simulink model "CC_dynamic_case"  (R2020b)
settings: Solver=VariableStepAuto  StartTime=0.0  StopTime=3600*2000  RelTol=1e-3
undefined symbols (not defined in the file or in its folder): Batt, BatteryCback, BatteryLoadFcn, gcbh, I_charge, I_discharge, Q, sps_rtmsupport
libraries: simulink x6, powerlib x5
settings Model: SimulationMode=rapid-accelerator  Creator=JIAHANG001  LastModifiedBy=jiahang001
settings SFSimCC: CustomCodeUndefinedFunction=UseInterfaceOnly

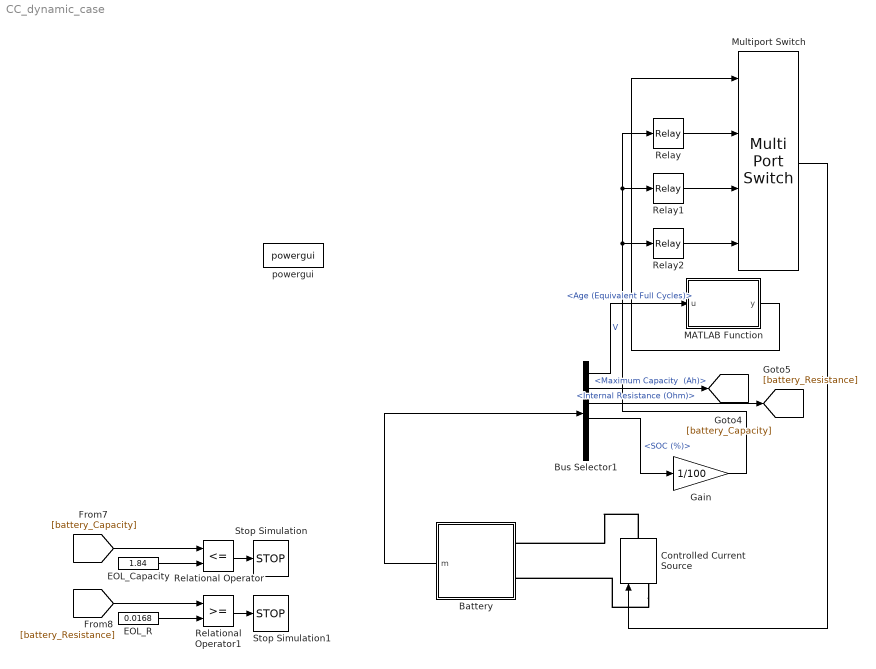
== system CC_dynamic_case ==
  Battery : Subsystem  AncestorBlock=electricdrivelib/Extra Sources/Battery  DialogController=POWERSYS.PowerSysDialog  LoadFcn=sps_rtmsupport('LoadFcn',gcbh); BatteryLoadFcn(gcb)  InitFcn=BatteryCback(gcb,1)  StartFcn=sps_rtmsupport('StartFcn',gcbh);  StopFcn=sps_rtmsupport('StopFcn',gcbh);  mask(Battery){BatType=Lithium-Ion, ShowTempParam=off, ThermalPreset=3.3V  2.3Ah  (LiFePO4), ShowAgeParam=on, NomV=3.3, NomQ=2.3, SOC=100, Batt_Tr=30, PresetModel=off, MaxQ=2.3, MinV=2.475, FullV=3.748, Dis_rate=2.3, R=0.014, Normal_OP=2.25, expZone=[3.4788       0.113], current=[0.15 1.3 3.25], Units=Ampere-hour, Tci=25, NomT=25, T2=0, MaxQ2=2.208, FullV2=3.45, Normal_OP2=2.85, expZone2=[3.22       0.015], Rca=0.6, ti=1000, Dp=0, Neq0=0, Tsim=60, Ta1=25, Qeol=2.3*0.8, Reol=0.014*1.2, Char_age=[2.3, 4.3], Dis_age=[2.3, 11.7], N1=1000, N2=1200, N3=400, N4=500, Ta2=45, N5=950}
      mask prompts: BatType "Type:"; ShowTempParam "Simulate temperature effects"; ThermalPreset "Use a preset battery:"; ShowAgeParam "Simulate aging effects"; NomV "Nominal voltage (V)"; NomQ "Rated capacity (Ah)"; SOC "Initial state-of-charge (%)"; Batt_Tr "Battery response time (s)"; PresetModel "Determined from the nominal parameters of the battery"; MaxQ "Maximum capacity (Ah)"; MinV "Cut-off Voltage (V)"; FullV "Fully charged voltage (V)"; Dis_rate "Nominal discharge current (A)"; R "Internal resistance (Ohms)"; Normal_OP "Capacity (Ah) at nominal voltage"; expZone "Exponential zone [Voltage (V), Capacity (Ah)]"; current "Discharge current [i1, i2, i3,...] (A)"; Tci "Initial cell temperature (deg. C)"; NomT "Nominal ambient temperature T1 (deg. C)"; T2 "Second ambient temperature T2 (deg. C)"; MaxQ2 "Maximum capacity (Ah)"; FullV2 "Initial discharge voltage (V)"; Normal_OP2 "Voltage at 90% maximum capacity (V)"; expZone2 "Exponential zone [Voltage (V), Capacity (Ah)]"; Rca "Thermal resistance, cell-to-ambient (deg. C/W)"; ti "Thermal time constant, cell-to-ambient (s)"; Dp "Heat loss difference [charge vs. discharge] (W)"; Neq0 "Initial battery age (Equivalent full cycles)"; Tsim "Aging model sampling time (s)"; Ta1 "Ambient temperature Ta1 (deg. C)"; Qeol "Capacity at EOL (End Of Life) (Ah)"; Reol "Internal resistance at EOL (Ohms)"; Char_age "Charge current (nominal, maximum) [Ic (A), Icmax (A)]"; Dis_age "Discharge current (nominal, maximum) [Id (A), Idmax (A)]"; N1 "Cycle life at 100 % DOD, Ic and Id (Cycles)"; N2 "Cycle life at 25 % DOD, Ic and Id (Cycles)"; N3 "Cycle life at 100 % DOD, Ic and Idmax (Cycles)"; N4 "Cycle life at 100 % DOD, Icmax and Id (Cycles)"; Ta2 "Ambient temperature Ta2 (deg. C)"; N5 "Cycle life at 100 % DOD, Ic and Id (Cycles)"
      mask help: Implements a generic battery model for most popular battery types. Temperature and aging (due to cycling) effects can be specified for Lithium-Ion battery type.
      mask init:
      | block = gcb;
      | BatteryCback(block,3)
      | [Batt BT, WantBlockChoice, Ts] = BatteryParam(NomV,NomQ,MaxQ,MinV,FullV,Dis_rate,R,Normal_OP,expZone,block,0);
      | powericon('SetInternalModels','set',block,WantBlockChoice);
      | BatteryCback(block,1);
      settings: CopyFcn=sps_rtmsupport('CopyFcn',gcbh);  DeleteFcn=sps_rtmsupport('DeleteFcn',gcbh);  UndoDeleteFcn=sps_rtmsupport('UndoDeleteFcn',gcbh);  ModelCloseFcn=sps_rtmsupport('ModelCloseFcn',gcbh);  PreSaveFcn=sps_rtmsupport('PreSaveFcn',gcbh);  PostSaveFcn=sps_rtmsupport('PostSaveFcn',gcbh);  NameChangeFcn=sps_rtmsupport('NameChangeFcn',gcbh);  PreCopyFcn=sps_rtmsupport('PreCopyFcn',gcbh);  OpenFcn=sps_rtmsupport('OpenFcn',gcbh, [1,2,3,4,9,18]);  CloseFcn=sps_rtmsupport('CloseFcn',gcbh);  PreDeleteFcn=sps_rtmsupport('PreDeleteFcn',gcbh);
      mask Help: helpview(psbhelp)
      mask TypeOptions BatType: Lead-Acid | Lithium-Ion | Nickel-Cadmium | Nickel-Metal-Hydride
      mask Callback BatType: BatteryCback(gcb,1)
      mask Callback ShowTempParam: BatteryCback(gcb,1)
      mask TypeOptions ThermalPreset: no | 3.3V  2.3Ah  (LiFePO4) | 3.6V  2050mAh   (LiCoO2) | 3.6V  2.0Ah | 3.6V  3.6Ah  (LiNiO2) | 3.6V  4.5Ah | 3.6V  48Ah  (LiNiO2) | 3.7V  4.4Ah | 7.4V  5.4Ah  (LiCoO2) | 11.1V  6600mAh  (LiCoO2) | 12.8V  40Ah  (LiFeMgPO4)
      mask Callback ThermalPreset: BatteryCback(gcb,4)
      mask Callback ShowAgeParam: BatteryCback(gcb,1)
      mask Callback PresetModel: BatteryCback(gcb,1)
      mask TypeOptions Units: Ampere-hour | Time
      mask Callback ti: sps_rtmsupport('parametereditingmodes',gcbh, [1,2,3,4,9,18]);
      mask DialogControl ParameterTabVar0 Prompt: Parameters
      mask DialogControl Tempcontainer Prompt: Temperature
      mask DialogControl Agecontainer Prompt: Aging
      mask DialogControl ParameterTabVar01 Prompt: Discharge
      mask DialogControl Container9 Prompt: Display characteristics
      mask DialogControl PlotButton Prompt: Plot
      mask DialogControl PlotButton Callback: BatteryCback(gcb,0)
      mask DialogControl Temperature Prompt: Temperature
      mask DialogControl Container7 Prompt: Discharge parameters at T2
      mask DialogControl Container8 Prompt: Thermal response and Heat loss
      mask DialogControl Aging Prompt: Aging
      mask DialogControl Container16 Prompt: Aging characteristics at ambient temperature Ta1
      mask DialogControl Container13 Prompt: Aging characteristics at ambient temperature Ta2
      mask Display:
      | patch([BT.X1 BT.X1m],[BT.Y1 BT.Y1m],BT.color1);
      | patch(BT.X3,BT.Y3,BT.color2);
      | plot([BT.X1 BT.X1m BT.X2 BT.X2m BT.X3 BT.X4],[BT.Y1 BT.Y1m BT.Y2 BT.Y2m BT.Y3 BT.Y4]);
      | plot(-100,-60,60,50,[BT.X(1) BT.X(1)],[BT.bas BT.haut],[BT.X(2) BT.X(2)],[BT.haut BT.bas],BT.dim_Xsin,4*sin(BT.dim_sin)+BT.haut,BT.dim_Xsin,-4*sin(BT.dim_sin)+BT.haut,BT.dim_Xsin,-4*sin(BT.dim_sin)+BT.bas,BT.dim_Xtop,sin(BT.dim_top)+BT.haut+4,BT.dim_Xtop,-sin(BT.dim_top)+BT.haut+4,BT.dim_Xtop,-sin(BT.dim_top)+BT.haut,[BT.TopX(2),BT.TopX(2)],[BT.haut,BT.haut+4],[BT.TopX(1),BT.TopX(1)],[BT.haut+4,BT.haut]);plot(BT.dim_Xsin,-5*sin(BT.dim_sin)+20);
      | port_label('lconn',1,'+');
      | port_label('lconn',2,'_');
      | color('blue');
      | port_label('output',1,'m');
      | 
      | if Batt.sel_T
      |     port_label('input',1,'Ta');
      | end
  Bus Selector1 : BusSelector  OutputSignals="Age (Equivalent Full Cycles),Maximum Capacity  (Ah),Internal Resistance (Ohm),SOC (%),Current (A),Voltage (V)"
  Controlled Current Source : powerlib/Electrical Sources/Controlled Current Source  Initialize=on  Source_Type=AC  Amplitude=0  Phase=0  Frequency=0  Measurements=None
  EOL_Capacity : Constant  Value=1.84
  EOL_R : Constant  Value=0.0168
  Gain : Gain  Gain=1/100
  MATLAB Function : MATLAB Function  TreatAsAtomicUnit=on
  Multiport Switch : MultiPortSwitch  DataPortOrder=Specify indices  DataPortIndices={400,800}  DataPortForDefault=Additional data port
  Relational Operator : RelationalOperator  Operator=<=  OutDataTypeStr=boolean  RndMeth=Simplest
  Relational Operator1 : RelationalOperator  OutDataTypeStr=boolean  RndMeth=Simplest
  Relay : Relay  OnSwitchValue=40/100  OffSwitchValue=1/100  OnOutputValue=-I_discharge(2)  OffOutputValue=I_charge(2)
  Relay1 : Relay  OnSwitchValue=60/100  OffSwitchValue=1/100  OnOutputValue=-I_discharge(2)  OffOutputValue=I_charge(2)
  Relay2 : Relay  OnSwitchValue=80/100  OffSwitchValue=20/100  OnOutputValue=-I_discharge(2)  OffOutputValue=I_charge(2)
  Stop Simulation : Stop
  Stop Simulation1 : Stop
  powergui : powerlib/powergui  SimulationMode=Discrete  SampleTime=0.05  frequency=60  Iterations=50  frequencyindice=0  Pbase=100e6  ErrMax=1e-4  UnitsV=kV  UnitsW=MW  buscounter=0  FunctionMessages=off  echomessages=off  EnableUseOfTLC=off  CurrentSourceSwitches=on  DisableSnubberDevices=off  DisableRonSwitches=off  DisableVfSwitches=off  DisplayEquations=off  AutomaticDiscreteSolvers=off  SolverType=Tustin  Interpol=off  ExternalGateDelay=off  methode=off  Ts=0  x0status=blocks  SPID=off  SwTol=0  HookPort=off  NonlinearTolerance=1e-4  nMaxIteration=100  ContinueOnMaxIteration=off  RestoreLinks=warning  ResistiveCurrentMeasurement=off  Frange=[0:2:500]  Ylog=off  Xlog=on  ShowGrid=off  save=off  variable=ZData  structure=0  ZoomFFT=on  StartTime=0.0  cycles=1  DisplayStyle=1  fundamental=60  FreqAxis=off  MaxFrequency=1000  frequencyindicesteady=1  RmsSteady=1  display=off
  wires:
  EOL_Capacity/1 -> Relational Operator/2
  [battery_Resistance] -> Relational Operator1/1
  Relational Operator/1 -> Stop Simulation/1
  Relational Operator1/1 -> Stop Simulation1/1
  [battery_Capacity] -> Relational Operator/1
  EOL_R/1 -> Relational Operator1/2
  Bus Selector1/3 -> [battery_Resistance]  "<Internal Resistance (Ohm)>"
  Bus Selector1/2 -> [battery_Capacity]  "<Maximum Capacity  (Ah)>"
  Bus Selector1/4 -> Gain/1  "<SOC (%)>"
  Battery/1(m) -> Bus Selector1/1
  MATLAB Function/1(y) -> Multiport Switch/1
  Bus Selector1/1 -> MATLAB Function/1(u)  "<Age (Equivalent Full Cycles)>"
  Relay2/1 -> Multiport Switch/4
  Relay1/1 -> Multiport Switch/3
  Relay/1 -> Multiport Switch/2
  Multiport Switch/1 -> Controlled Current Source/1
  Gain/1 -> Relay/1, Relay1/1, Relay2/1  "V"
  connections:
  Controlled Current Source/RConn1 -- Battery/LConn1
  Controlled Current Source/LConn1 -- Battery/LConn2

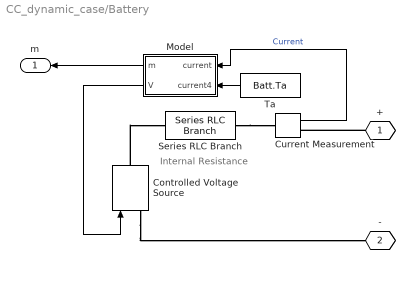
== system CC_dynamic_case/Battery ==
  note: Internal Resistance
  Controlled Voltage Source : powerlib/Electrical Sources/Controlled Voltage Source  Initialize=on  Source_Type=AC  Amplitude=0  Phase=0  Frequency=0  Measurements=None
  Current Measurement : powerlib/Measurements/Current Measurement  PhasorSimulation=off  OutputType=Complex  PSBequivalent=0
  Model : Subsystem  AncestorBlock=spsBatteryModel/Continuous thermal aging
  Series RLC Branch : powerlib/Elements/Series RLC Branch  LConnTagsString=__new0  RConnTagsString=__new0  BranchType=R  Resistance=Batt.R  Inductance=1e-3  SetiL0=off  InitialCurrent=0  Capacitance=1e-6  Setx0=off  InitialVoltage=0  Measurements=None
  Ta : Constant  Value=Batt.Ta
  + : PMIOPort  Tag=PMCPort  Side=Left
  - : PMIOPort  Tag=PMCPort  Port=2  Side=Left
  m : Outport  VectorParamsAs1DForOutWhenUnconnected=off
  wires:
  Ta/1 -> Model/2(current4)
  Model/2(V) -> Controlled Voltage Source/1
  Model/1(m) -> m/1
  Current Measurement/1 -> Model/1(current)  "Current"
  connections:
  +/RConn1 -- Current Measurement/RConn1
  Controlled Voltage Source/LConn1 -- -/RConn1
  Controlled Voltage Source/RConn1 -- Series RLC Branch/LConn1
  Series RLC Branch/RConn1 -- Current Measurement/LConn1

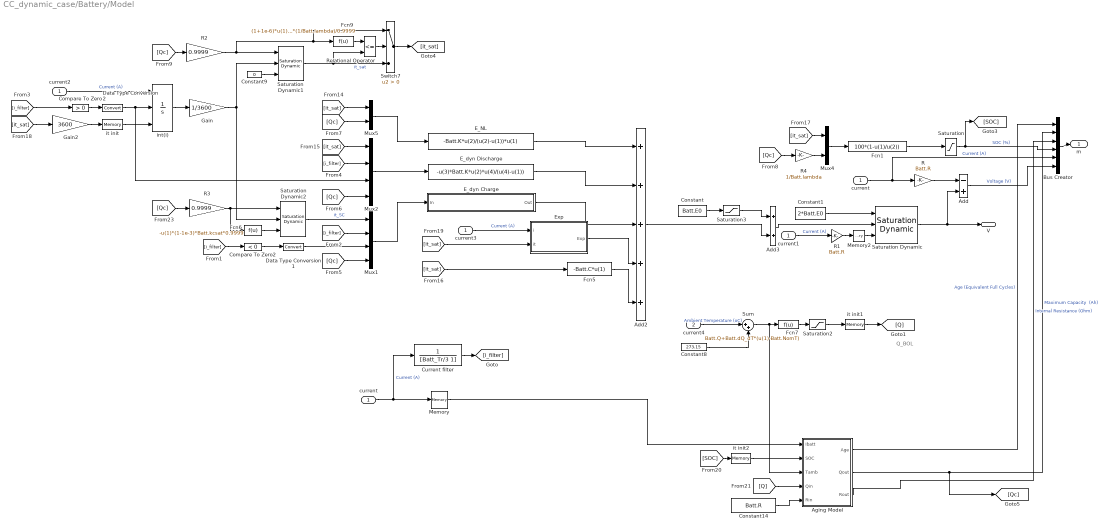
== system CC_dynamic_case/Battery/Model ==
  note: Q_BOL
  current : Inport
  current4 : Inport  Port=2
  Add : Sum  Inputs=-+
  Add2 : Sum  Inputs=+++++
  Add3 : Sum
  Aging Model : Subsystem  AncestorBlock=spsBatteryModel/Aging Model
  Bus Creator : BusCreator  Inputs=6
  Compare To Zero : simulink/Logic and Bit Operations/Compare To Zero  relop=>  OutDataTypeStr=uint8
  Compare To Zero2 : simulink/Logic and Bit Operations/Compare To Zero  relop=<  OutDataTypeStr=uint8
  Constant : Constant  Value=Batt.E0
  Constant1 : Constant  Value=2*Batt.E0
  Constant14 : Constant  Value=Batt.R
  Constant8 : Constant  Value=273.15
  Constant9 : Constant  Value=0
  Current filter : TransferFcn  Denominator=[Batt_Tr/3 1]
  Data Type Conversion1 : DataTypeConversion
  Data Type Conversion2 : DataTypeConversion
  E_NL : Fcn  Expr=-Batt.K*u(2)/(u(2)-u(1))*u(1)
  E_dyn Charge : Subsystem
  E_dyn Discharge : Fcn  Expr=-u(3)*Batt.K*u(2)*u(4)/(u(4)-u(1))
  Exp : Subsystem
  Fcn1 : Fcn  Expr=100*(1-u(1)/u(2))
  Fcn5 : Fcn  Expr=-Batt.C*u(1)
  Fcn6 : Fcn  Expr=-u(1)*(1-1e-3)*Batt.kcsat*0.9999
  Fcn7 : Fcn  Expr=Batt.Q+Batt.dQ_dT*(u(1)-Batt.NomT)
  Fcn9 : Fcn  Expr=(1+1e-6)*u(1)*(1/Batt.lambda)/0.9999
  Gain : Gain  Gain=1/3600
  Gain2 : Gain  Gain=3600
  Memory : Memory
  Memory2 : Memory  InheritSampleTime=on
  Mux1 : Mux
  Mux2 : Mux
  Mux4 : Mux  Inputs=2
  Mux5 : Mux  Inputs=2
  R : Gain  Gain=Batt.R
  R1 : Gain  Gain=Batt.R
  R2 : Gain  Gain=0.9999
  R3 : Gain  Gain=0.9999
  R4 : Gain  Gain=1/Batt.lambda
  Relational Operator : RelationalOperator  Operator=<=  RndMeth=Simplest
  Saturation : Saturate  UpperLimit=100  LowerLimit=0
  Saturation Dynamic : simulink/Discontinuities/Saturation Dynamic  OutMin=[]  OutMax=[]  OutDataTypeStr=Inherit: Same as second input  OutDataType=sfix(16)  OutScaling=2^-10  DoSatur=off
  Saturation Dynamic1 : simulink/Discontinuities/Saturation Dynamic  OutMin=[]  OutMax=[]  OutDataTypeStr=Inherit: Same as second input  OutDataType=sfix(16)  OutScaling=2^-10  DoSatur=off
  Saturation Dynamic2 : simulink/Discontinuities/Saturation Dynamic  OutMin=[]  OutMax=[]  OutDataTypeStr=Inherit: Same as second input  OutDataType=sfix(16)  OutScaling=2^-10  DoSatur=off
  Saturation2 : Saturate  UpperLimit=max(NomQ,Batt.Q)  LowerLimit=0
  Saturation3 : Saturate  UpperLimit=Batt.Va-Batt.dE_dT*(Batt.Tci-Batt.NomT)-Batt.A  LowerLimit=-inf
  Sum : Sum  Inputs=|++
  Switch7 : Switch  Criteria=u2 > Threshold
  "current " : InportShadow
  current1 : InportShadow
  current2 : InportShadow
  current3 : InportShadow
  int(i) : Integrator  ExternalReset=rising  InitialConditionSource=external  InitialCondition=(1-SOC/100)*Q*3600  LimitOutput=on  UpperSaturationLimit=Batt.Qmax*3600
  it init : Memory  InitialCondition=(1-SOC/100)*Batt.Q*(1/Batt.lambda)*3600
  it init1 : Memory  InitialCondition=Batt.Q
  it init2 : Memory  InitialCondition=SOC
  m : Outport  VectorParamsAs1DForOutWhenUnconnected=off
  V : Outport  Port=2  VectorParamsAs1DForOutWhenUnconnected=off
  wires:
  R1/1 -> Memory2/1
  current1/1 -> R1/1  "Current (A)"
  Memory2/1 -> Saturation Dynamic/3
  Add/1 -> Bus Creator/6  "Voltage (V)"
  current/1 -> R/1, Bus Creator/5  "Current (A)"
  int(i)/1 -> Gain/1
  Fcn1/1 -> Saturation/1
  R/1 -> Add/1
  Bus Creator/1 -> m/1
  Mux2/1 -> E_dyn Discharge/1
  Constant/1 -> Saturation3/1
  Mux1/1 -> E_dyn Charge/1(In)
  it init/1 -> int(i)/3
  Compare To Zero/1 -> Data Type Conversion2/1
  Compare To Zero2/1 -> Data Type Conversion1/1
  Data Type Conversion2/1 -> Mux2/3, int(i)/2
  Gain2/1 -> it init/1
  Exp/1(Exp) -> Add2/4
  Data Type Conversion1/1 -> Mux1/3
  Saturation Dynamic2/1 -> Mux1/1  "it_SC"
  Constant1/1 -> Saturation Dynamic/1
  Add3/1 -> Saturation Dynamic/2
  E_dyn Discharge/1 -> Add2/2
  E_NL/1 -> Add2/1
  Memory/1 -> Aging Model/1(Ibatt)
  E_dyn Charge/1(Out) -> Add2/3
  Fcn5/1 -> Add2/5
  current4/1 -> Sum/1  "Ambient Temperature (oC)"
  Constant8/1 -> Sum/2
  Mux4/1 -> Fcn1/1
  Mux5/1 -> E_NL/1
  Fcn6/1 -> Saturation Dynamic2/3
  Sum/1 -> Aging Model/3(Tamb), Fcn7/1
  Fcn7/1 -> Saturation2/1
  Saturation3/1 -> Add3/1
  Saturation2/1 -> it init1/1
  current2/1 -> int(i)/1  "Current (A)"
  current3/1 -> Exp/1(i)  "Current (A)"
  "current "/1 -> Memory/1, Current filter/1  "Current (A)"
  Current filter/1 -> [i_filter]
  [i_filter] -> Compare To Zero2/1
  [i_filter] -> Mux1/2
  [i_filter] -> Compare To Zero/1
  [i_filter] -> Mux2/2
  it init1/1 -> [Q]
  [Qc] -> Mux1/4
  [Qc] -> Mux2/4
  [Qc] -> R4/1
  [Qc] -> R2/1
  [it_sat] -> Mux5/1
  [it_sat] -> Mux2/1
  [it_sat] -> Fcn5/1
  [it_sat] -> Mux4/1
  [it_sat] -> Gain2/1
  [it_sat] -> Exp/2(it)
  [Qc] -> R3/1
  R3/1 -> Fcn6/1, Saturation Dynamic2/1
  Add2/1 -> Add3/2
  R4/1 -> Mux4/2
  Saturation/1 -> [SOC], Bus Creator/4  "SOC (%)"
  Saturation Dynamic/1 -> V/1, Add/2
  [Qc] -> Mux5/2
  [SOC] -> it init2/1
  [Q] -> Aging Model/4(Qin)
  Aging Model/2(Qout) -> Bus Creator/2, [Qc]  "Maximum Capacity  (Ah)"
  Constant14/1 -> Aging Model/5(Rin)
  Aging Model/3(Rout) -> Bus Creator/3  "Internal Resistance (Ohm)"
  Aging Model/1(Age) -> Bus Creator/1  "Age (Equivalent Full Cycles)"
  it init2/1 -> Aging Model/2(SOC)
  Gain/1 -> Saturation Dynamic1/2, Saturation Dynamic2/2
  Constant9/1 -> Saturation Dynamic1/3
  Saturation Dynamic1/1 -> Relational Operator/2, Switch7/3  "it_sat"
  R2/1 -> Switch7/1, Fcn9/1, Saturation Dynamic1/1
  Switch7/1 -> [it_sat]
  Fcn9/1 -> Relational Operator/1
  Relational Operator/1 -> Switch7/2

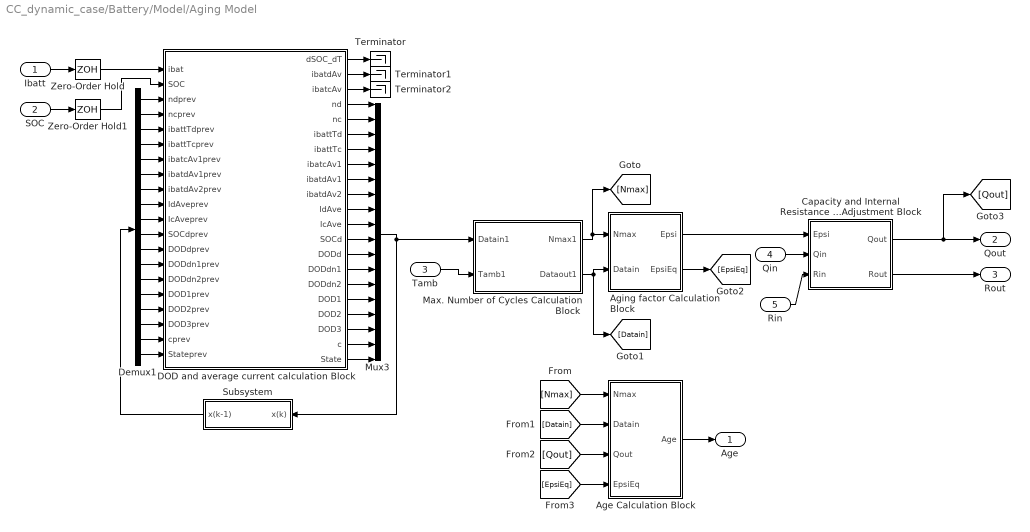
== system CC_dynamic_case/Battery/Model/Aging Model ==
  Ibatt : Inport
  SOC : Inport  Port=2
  Tamb : Inport  Port=3
  Qin : Inport  Port=4
  Rin : Inport  Port=5
  Age Calculation Block : Subsystem
  Aging factor Calculation Block : Subsystem
  Capacity and Internal Resistance Adjustment Block : Subsystem
  DOD and average current calculation Block : MATLAB Function  TreatAsAtomicUnit=on
  Demux1 : Demux  Outputs=18
      settings: DisplayOption=none
  Max. Number of Cycles Calculation Block : Subsystem
  Mux3 : Mux  Inputs=18
  Subsystem : Subsystem
  Terminator : Terminator
  Terminator1 : Terminator
  Terminator2 : Terminator
  Zero-Order Hold : ZeroOrderHold  SampleTime=Batt.Tsim
  Zero-Order Hold1 : ZeroOrderHold  SampleTime=Batt.Tsim
  Age : Outport  VectorParamsAs1DForOutWhenUnconnected=off
  Qout : Outport  Port=2  VectorParamsAs1DForOutWhenUnconnected=off
  Rout : Outport  Port=3  VectorParamsAs1DForOutWhenUnconnected=off
  wires:
  [EpsiEq] -> Age Calculation Block/4(EpsiEq)
  [Qout] -> Age Calculation Block/3(Qout)
  [Datain] -> Age Calculation Block/2(Datain)
  Aging factor Calculation Block/2(EpsiEq) -> [EpsiEq]
  [Nmax] -> Age Calculation Block/1(Nmax)
  Age Calculation Block/1(Age) -> Age/1
  Capacity and Internal Resistance Adjustment Block/1(Qout) -> Qout/1, [Qout]
  Mux3/1 -> Max. Number of Cycles Calculation Block/1(Datain1), Subsystem/1(x(k))
  Aging factor Calculation Block/1(Epsi) -> Capacity and Internal Resistance Adjustment Block/1(Epsi)
  Capacity and Internal Resistance Adjustment Block/2(Rout) -> Rout/1
  Rin/1 -> Capacity and Internal Resistance Adjustment Block/3(Rin)
  Qin/1 -> Capacity and Internal Resistance Adjustment Block/2(Qin)
  Tamb/1 -> Max. Number of Cycles Calculation Block/2(Tamb1)
  DOD and average current calculation Block/9(ibatdAv1) -> Mux3/6
  Demux1/10 -> DOD and average current calculation Block/12(SOCdprev)
  Demux1/3 -> DOD and average current calculation Block/5(ibattTdprev)
  Demux1/13 -> DOD and average current calculation Block/15(DODdn2prev)
  DOD and average current calculation Block/4(nd) -> Mux3/1
  DOD and average current calculation Block/16(DODdn2) -> Mux3/13
  Demux1/6 -> DOD and average current calculation Block/8(ibatdAv1prev)
  Demux1/12 -> DOD and average current calculation Block/14(DODdn1prev)
  Demux1/9 -> DOD and average current calculation Block/11(IcAveprev)
  Demux1/16 -> DOD and average current calculation Block/18(DOD3prev)
  Demux1/17 -> DOD and average current calculation Block/19(cprev)
  DOD and average current calculation Block/5(nc) -> Mux3/2
  DOD and average current calculation Block/15(DODdn1) -> Mux3/12
  DOD and average current calculation Block/21(State) -> Mux3/18
  DOD and average current calculation Block/13(SOCd) -> Mux3/10
  Demux1/18 -> DOD and average current calculation Block/20(Stateprev)
  DOD and average current calculation Block/20(c) -> Mux3/17
  Demux1/11 -> DOD and average current calculation Block/13(DODdprev)
  DOD and average current calculation Block/6(ibattTd) -> Mux3/3
  Demux1/15 -> DOD and average current calculation Block/17(DOD2prev)
  Demux1/7 -> DOD and average current calculation Block/9(ibatdAv2prev)
  DOD and average current calculation Block/14(DODd) -> Mux3/11
  DOD and average current calculation Block/10(ibatdAv2) -> Mux3/7
  DOD and average current calculation Block/19(DOD3) -> Mux3/16
  DOD and average current calculation Block/11(IdAve) -> Mux3/8
  DOD and average current calculation Block/7(ibattTc) -> Mux3/4
  Demux1/4 -> DOD and average current calculation Block/6(ibattTcprev)
  DOD and average current calculation Block/8(ibatcAv1) -> Mux3/5
  Demux1/14 -> DOD and average current calculation Block/16(DOD1prev)
  Demux1/8 -> DOD and average current calculation Block/10(IdAveprev)
  DOD and average current calculation Block/17(DOD1) -> Mux3/14
  DOD and average current calculation Block/12(IcAve) -> Mux3/9
  DOD and average current calculation Block/18(DOD2) -> Mux3/15
  Demux1/1 -> DOD and average current calculation Block/3(ndprev)
  Subsystem/1(x(k-1)) -> Demux1/1
  Demux1/2 -> DOD and average current calculation Block/4(ncprev)
  DOD and average current calculation Block/1(dSOC_dT) -> Terminator/1
  DOD and average current calculation Block/3(ibatcAv) -> Terminator2/1
  DOD and average current calculation Block/2(ibatdAv) -> Terminator1/1
  Demux1/5 -> DOD and average current calculation Block/7(ibatcAv1prev)
  Max. Number of Cycles Calculation Block/1(Nmax1) -> Aging factor Calculation Block/1(Nmax), [Nmax]
  Max. Number of Cycles Calculation Block/2(Dataout1) -> Aging factor Calculation Block/2(Datain), [Datain]
  Ibatt/1 -> Zero-Order Hold/1
  SOC/1 -> Zero-Order Hold1/1
  Zero-Order Hold/1 -> DOD and average current calculation Block/1(ibat)
  Zero-Order Hold1/1 -> DOD and average current calculation Block/2(SOC)

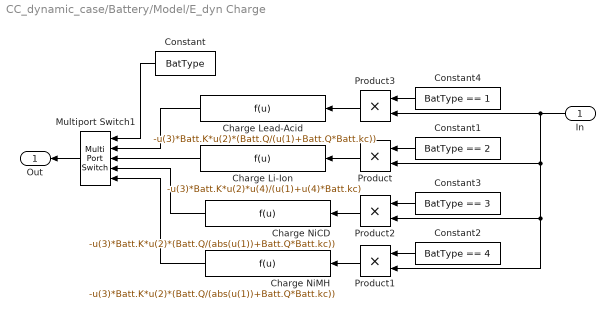
== system CC_dynamic_case/Battery/Model/E_dyn Charge ==
  In : Inport
  Charge Lead-Acid : Fcn  Expr=-u(3)*Batt.K*u(2)*(Batt.Q/(u(1)+Batt.Q*Batt.kc))
  Charge Li-Ion : Fcn  Expr=-u(3)*Batt.K*u(2)*u(4)/(u(1)+u(4)*Batt.kc)
  Charge NiCD : Fcn  Expr=-u(3)*Batt.K*u(2)*(Batt.Q/(abs(u(1))+Batt.Q*Batt.kc))
  Charge NiMH : Fcn  Expr=-u(3)*Batt.K*u(2)*(Batt.Q/(abs(u(1))+Batt.Q*Batt.kc))
  Constant : Constant  Value=BatType
  Constant1 : Constant  Value=BatType == 2  OutDataTypeStr=double
  Constant2 : Constant  Value=BatType == 4  OutDataTypeStr=double
  Constant3 : Constant  Value=BatType == 3  OutDataTypeStr=double
  Constant4 : Constant  Value=BatType == 1  OutDataTypeStr=double
  Multiport Switch1 : MultiPortSwitch  Inputs=4
  Product{,1..3} (4 alike) : Product  RndMeth=Zero
  Out : Outport  VectorParamsAs1DForOutWhenUnconnected=off
  wires:
  Multiport Switch1/1 -> Out/1
  Charge Li-Ion/1 -> Multiport Switch1/3
  Charge NiMH/1 -> Multiport Switch1/5
  Charge NiCD/1 -> Multiport Switch1/4
  Charge Lead-Acid/1 -> Multiport Switch1/2
  Constant/1 -> Multiport Switch1/1
  In/1 -> Product3/2, Product/2, Product1/2, Product2/2
  Product/1 -> Charge Li-Ion/1
  Constant1/1 -> Product/1
  Product1/1 -> Charge NiMH/1
  Constant2/1 -> Product1/1
  Product2/1 -> Charge NiCD/1
  Constant3/1 -> Product2/1
  Product3/1 -> Charge Lead-Acid/1
  Constant4/1 -> Product3/1

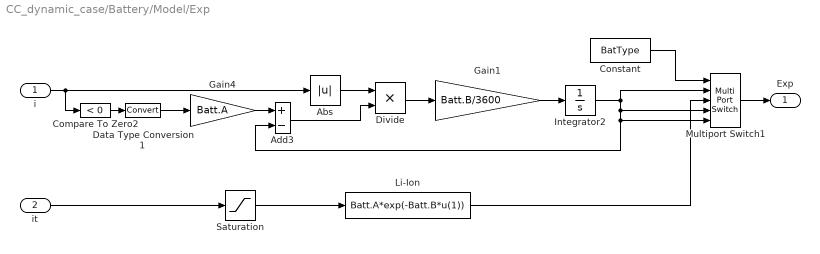
== system CC_dynamic_case/Battery/Model/Exp ==
  i : Inport
  it : Inport  Port=2
  Abs : Abs
  Add3 : Sum  Inputs=+-
  Compare To Zero2 : simulink/Logic and Bit Operations/Compare To Zero  relop=<  OutDataTypeStr=uint8
  Constant : Constant  Value=BatType
  Data Type Conversion1 : DataTypeConversion
  Divide : Product  Inputs=**
  Gain1 : Gain  Gain=Batt.B/3600
  Gain4 : Gain  Gain=Batt.A
  Integrator2 : Integrator  InitialCondition=Batt.A*exp(-Batt.B*(1-SOC/100)*Batt.Q)
  Li-Ion : Fcn  Expr=Batt.A*exp(-Batt.B*u(1))
  Multiport Switch1 : MultiPortSwitch  Inputs=4
  Saturation : Saturate  UpperLimit=Batt.Qmax*(1/Batt.lambda)  LowerLimit=-inf
  Exp : Outport  VectorParamsAs1DForOutWhenUnconnected=off
  wires:
  Integrator2/1 -> Multiport Switch1/2, Multiport Switch1/4, Add3/2, Multiport Switch1/5
  Gain4/1 -> Add3/1
  Divide/1 -> Gain1/1
  Abs/1 -> Divide/1
  Add3/1 -> Divide/2
  Gain1/1 -> Integrator2/1
  i/1 -> Abs/1, Compare To Zero2/1
  Constant/1 -> Multiport Switch1/1
  it/1 -> Saturation/1
  Li-Ion/1 -> Multiport Switch1/3
  Multiport Switch1/1 -> Exp/1
  Compare To Zero2/1 -> Data Type Conversion1/1
  Data Type Conversion1/1 -> Gain4/1
  Saturation/1 -> Li-Ion/1

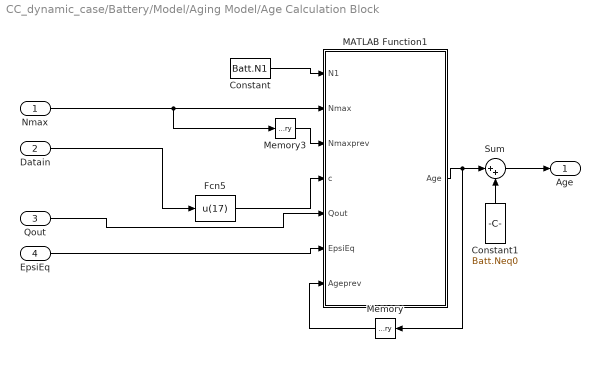
== system CC_dynamic_case/Battery/Model/Aging Model/Age Calculation Block ==
  Nmax : Inport
  Datain : Inport  Port=2
  Qout : Inport  Port=3
  EpsiEq : Inport  Port=4
  Constant : Constant  Value=Batt.N1
  Constant1 : Constant  Value=Batt.Neq0
  Fcn5 : Fcn  Expr=u(17)
  MATLAB Function1 : MATLAB Function  TreatAsAtomicUnit=on
  Memory : Memory  InheritSampleTime=on
  Memory3 : Memory  InheritSampleTime=on
  Sum : Sum  Inputs=|++
  Age : Outport  VectorParamsAs1DForOutWhenUnconnected=off
  wires:
  Constant1/1 -> Sum/2
  Sum/1 -> Age/1
  EpsiEq/1 -> MATLAB Function1/6(EpsiEq)
  Qout/1 -> MATLAB Function1/5(Qout)
  MATLAB Function1/1(Age) -> Memory/1, Sum/1
  Memory3/1 -> MATLAB Function1/3(Nmaxprev)
  Nmax/1 -> MATLAB Function1/2(Nmax), Memory3/1
  Datain/1 -> Fcn5/1
  Constant/1 -> MATLAB Function1/1(N1)
  Fcn5/1 -> MATLAB Function1/4(c)
  Memory/1 -> MATLAB Function1/7(Ageprev)

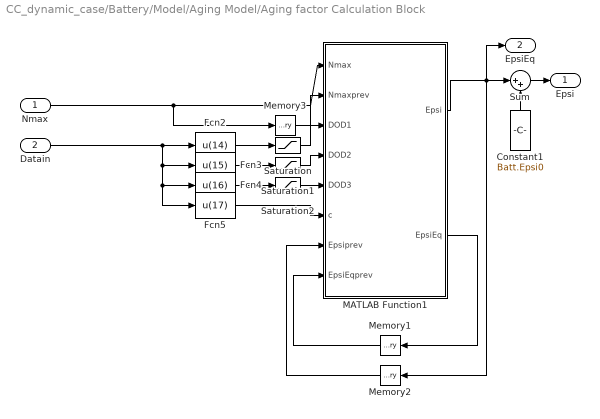
== system CC_dynamic_case/Battery/Model/Aging Model/Aging factor Calculation Block ==
  Nmax : Inport
  Datain : Inport  Port=2
  Constant1 : Constant  Value=Batt.Epsi0
  Fcn2 : Fcn  Expr=u(14)
  Fcn3 : Fcn  Expr=u(15)
  Fcn4 : Fcn  Expr=u(16)
  Fcn5 : Fcn  Expr=u(17)
  MATLAB Function1 : MATLAB Function  TreatAsAtomicUnit=on
  Memory1 : Memory  InheritSampleTime=on
  Memory2 : Memory  InheritSampleTime=on
  Memory3 : Memory  InheritSampleTime=on
  Saturation : Saturate  UpperLimit=inf  LowerLimit=0.01
  Saturation1 : Saturate  UpperLimit=inf  LowerLimit=0.01
  Saturation2 : Saturate  UpperLimit=inf  LowerLimit=0.01
  Sum : Sum  Inputs=|++
  Epsi : Outport  VectorParamsAs1DForOutWhenUnconnected=off
  EpsiEq : Outport  Port=2  VectorParamsAs1DForOutWhenUnconnected=off
  wires:
  Memory3/1 -> MATLAB Function1/2(Nmaxprev)
  MATLAB Function1/1(Epsi) -> Memory2/1, Sum/1, EpsiEq/1
  Nmax/1 -> MATLAB Function1/1(Nmax), Memory3/1
  Saturation2/1 -> MATLAB Function1/5(DOD3)
  Fcn2/1 -> Saturation/1
  Saturation1/1 -> MATLAB Function1/4(DOD2)
  Fcn4/1 -> Saturation2/1
  Fcn3/1 -> Saturation1/1
  Datain/1 -> Fcn2/1, Fcn3/1, Fcn5/1, Fcn4/1
  Memory2/1 -> MATLAB Function1/7(Epsiprev)
  Saturation/1 -> MATLAB Function1/3(DOD1)
  MATLAB Function1/2(EpsiEq) -> Memory1/1
  Memory1/1 -> MATLAB Function1/8(EpsiEqprev)
  Fcn5/1 -> MATLAB Function1/6(c)
  Sum/1 -> Epsi/1
  Constant1/1 -> Sum/2

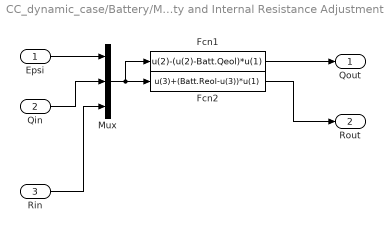
== system CC_dynamic_case/Battery/Model/Aging Model/Capacity and Internal Resistance Adjustment Block ==
  Epsi : Inport
  Qin : Inport  Port=2
  Rin : Inport  Port=3
  Fcn1 : Fcn  Expr=u(2)-(u(2)-Batt.Qeol)*u(1)
  Fcn2 : Fcn  Expr=u(3)+(Batt.Reol-u(3))*u(1)
  Mux : Mux  Inputs=3
  Qout : Outport  VectorParamsAs1DForOutWhenUnconnected=off
  Rout : Outport  Port=2  VectorParamsAs1DForOutWhenUnconnected=off
  wires:
  Fcn1/1 -> Qout/1
  Mux/1 -> Fcn1/1, Fcn2/1
  Fcn2/1 -> Rout/1
  Epsi/1 -> Mux/1
  Rin/1 -> Mux/3
  Qin/1 -> Mux/2

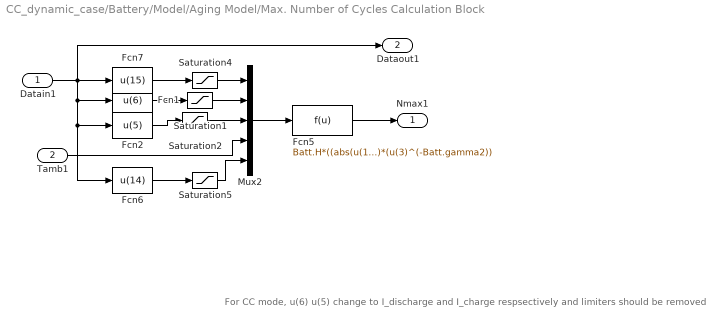
== system CC_dynamic_case/Battery/Model/Aging Model/Max. Number of Cycles Calculation Block ==
  note: For CC mode, u(6) u(5) change to I_discharge and I_charge respsectively and limiters should be removed
  Datain1 : Inport
  Tamb1 : Inport  Port=2
  Fcn1 : Fcn  Expr=u(6)
  Fcn2 : Fcn  Expr=u(5)
  Fcn5 : Fcn  Expr=Batt.H*((abs(u(1)-u(5))/100)^(-1))*exp(-Batt.phi*((1/Batt.Tref)-(1/u(4))))*(u(2)^(-Batt.gamma1))*(u(3)^(-Batt.gamma2))
  Fcn6 : Fcn  Expr=u(14)
  Fcn7 : Fcn  Expr=u(15)
  Mux2 : Mux  Inputs=5
  Saturation{1..2,4..5} (4 alike) : Saturate  UpperLimit=inf  LowerLimit=0.01
  Nmax1 : Outport  VectorParamsAs1DForOutWhenUnconnected=off
  Dataout1 : Outport  Port=2  VectorParamsAs1DForOutWhenUnconnected=off
  wires:
  Datain1/1 -> Fcn7/1, Fcn1/1, Fcn2/1, Fcn6/1, Dataout1/1
  Mux2/1 -> Fcn5/1
  Tamb1/1 -> Mux2/4
  Saturation4/1 -> Mux2/1
  Fcn7/1 -> Saturation4/1
  Fcn5/1 -> Nmax1/1
  Fcn6/1 -> Saturation5/1
  Saturation5/1 -> Mux2/5
  Saturation1/1 -> Mux2/2
  Fcn1/1 -> Saturation1/1
  Saturation2/1 -> Mux2/3
  Fcn2/1 -> Saturation2/1

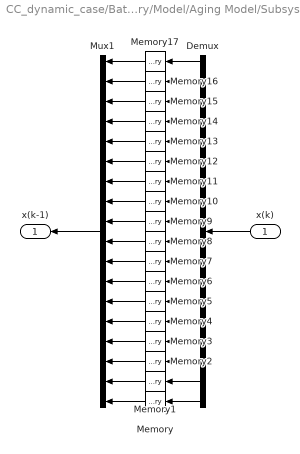
== system CC_dynamic_case/Battery/Model/Aging Model/Subsystem ==
  x(k) : Inport
  Demux : Demux  Outputs=18
      settings: DisplayOption=none
  Memory : Memory  InitialCondition=1  InheritSampleTime=on
  Memory{1..7,9..17} (16 alike) : Memory  InheritSampleTime=on
  Memory8 : Memory  InitialCondition=SOC  InheritSampleTime=on
  Mux1 : Mux  Inputs=18
  x(k-1) : Outport  VectorParamsAs1DForOutWhenUnconnected=off
  wires:
  Mux1/1 -> x(k-1)/1
  x(k)/1 -> Demux/1
  Demux/18 -> Memory/1
  Demux/17 -> Memory1/1
  Demux/16 -> Memory2/1
  Demux/15 -> Memory3/1
  Demux/14 -> Memory4/1
  Demux/13 -> Memory5/1
  Demux/12 -> Memory6/1
  Demux/11 -> Memory7/1
  Demux/10 -> Memory8/1
  Demux/9 -> Memory9/1
  Demux/8 -> Memory10/1
  Demux/7 -> Memory11/1
  Demux/6 -> Memory12/1
  Demux/5 -> Memory13/1
  Demux/4 -> Memory14/1
  Demux/3 -> Memory15/1
  Demux/2 -> Memory16/1
  Demux/1 -> Memory17/1
  Memory17/1 -> Mux1/1
  Memory15/1 -> Mux1/3
  Memory16/1 -> Mux1/2
  Memory14/1 -> Mux1/4
  Memory13/1 -> Mux1/5
  Memory12/1 -> Mux1/6
  Memory11/1 -> Mux1/7
  Memory10/1 -> Mux1/8
  Memory9/1 -> Mux1/9
  Memory8/1 -> Mux1/10
  Memory7/1 -> Mux1/11
  Memory6/1 -> Mux1/12
  Memory5/1 -> Mux1/13
  Memory4/1 -> Mux1/14
  Memory3/1 -> Mux1/15
  Memory2/1 -> Mux1/16
  Memory1/1 -> Mux1/17
  Memory/1 -> Mux1/18

== matlab function CC_dynamic_case/Battery/Model/Aging Model/Age Calculation Block/MATLAB Function1 ==
  data: N1 input; Nmax input; Nmaxprev input; c input; Qout input; EpsiEq input; Ageprev input; Age output
function Age = fcn(N1, Nmax, Nmaxprev,c,Qout,EpsiEq,Ageprev)
%#codegen
Age = Ageprev;
% Age = Neq0;

if(c>=3)
if (Nmax==Nmaxprev)
    Age = Ageprev;    
else 
    Age = EpsiEq*N1; % N1

%     if Qout>=2.3*0.91        
%         Age = EpsiEq*N1;
%     else
%         Age = EpsiEq*N1+EpsiEq*Nmax; % N1
%     end
    
end
end

== matlab function CC_dynamic_case/Battery/Model/Aging Model/Aging factor Calculation Block/MATLAB Function1 ==
  data: Nmax input; Epsi output; Nmaxprev input; DOD1 input; DOD2 input; DOD3 input; c input; Epsiprev input; EpsiEqprev input; EpsiEq output
function [Epsi,EpsiEq] = fcn(Nmax, Nmaxprev,DOD1,DOD2,DOD3,c,Epsiprev,EpsiEqprev)
%#codegen
 Epsi = Epsiprev;
 EpsiEq = EpsiEqprev;
 
if(c>=3)
if (Nmax==Nmaxprev)
    Epsi = Epsiprev;
    EpsiEq = EpsiEqprev;
    
else 
    Epsi = Epsiprev+(0.5/Nmax)*(1-(DOD3/DOD2))+(0.5/Nmax)*(1-(DOD1/DOD2));

end
end

== matlab function CC_dynamic_case/MATLAB Function ==
  data: u input; y output
function y = fcn(u)

if u>=800
	y=800;
elseif u>=400
    y=400;
else
    y=0;
end

end

== matlab function CC_dynamic_case/Battery/Model/Aging Model/DOD and average current calculation Block ==
  data: dSOC_dT output; ibatdAv output; ibatcAv output; ibat input; SOC input; ndprev input; ncprev input; ibattTdprev input; ibattTcprev input; ibatcAv1prev input; ibatdAv1prev input; ibatdAv2prev input; IdAveprev input; IcAveprev input; nd output; nc output; ibattTd output; ibattTc output; ibatcAv1 output; ibatdAv1 output; ibatdAv2 output; IdAve output; IcAve output; SOCdprev input; SOCd output; DODd output; DODdn1 output; DODdn2 output; DOD1 output; DOD2 output; DOD3 output; c output; DODdprev input; DODdn1prev input; DODdn2prev input; DOD1prev input; DOD2prev input; DOD3prev input; cprev input; Stateprev input; State output
function [dSOC_dT,ibatdAv,ibatcAv,nd,nc,ibattTd,ibattTc,ibatcAv1,ibatdAv1,ibatdAv2,IdAve,IcAve,SOCd,DODd,DODdn1,DODdn2,DOD1,DOD2,DOD3,c,State] = fcn(ibat,SOC,ndprev,ncprev,ibattTdprev,ibattTcprev,ibatcAv1prev,ibatdAv1prev,ibatdAv2prev,IdAveprev,IcAveprev,SOCdprev, DODdprev,DODdn1prev,DODdn2prev,DOD1prev, DOD2prev,DOD3prev,cprev,Stateprev)
%#codegen
DOD = 100 - SOCdprev; % original:100-SOC  possible:Q(n)/Q_BOL*100 no
dSOC_dT= (SOC-SOCdprev);
SOCd = SOC; % same output value
nd=ndprev+1;
nc=ncprev+1;
if(dSOC_dT <=0)
    s=0;
else
    s=1;
end
IdAve=IdAveprev;
IcAve=IcAveprev;
if(s==0)
ibattTd=ibattTdprev+abs(ibat);
ibatdAv =ibattTd/nd;
IdAve = ibatdAv;
ibattTc=0;
nc=0;
ibatcAv=0;
else
    ibattTd=0;
    nd=0;
    ibatdAv=0;
    ibattTc=ibattTcprev+abs(ibat);
    ibatcAv =ibattTc/nc;
    IcAve=ibatcAv;
end
sprev = Stateprev;
c=cprev;
if (s==sprev)
    DODdn2 = DODdn2prev;
    DODdn1 = DODdn1prev;
    DODd=DODdprev;
else
    DODd = DOD;
    c=cprev+1;
    DODdn2 = DODdn1prev;
    DODdn1 = DODdprev;
end
State=s;
ibatdAv2=ibatdAv2prev;
if(mod(c,2)==0)
    ibatdAv2=IdAveprev;
end
DOD1=DOD1prev;
DOD2=DOD2prev;
DOD3=DOD3prev;
ibatcAv1=ibatcAv1prev;
ibatdAv1=ibatdAv1prev;
if(mod(c,2)>0)
    DOD1=DODd;
    DOD2=DODdn1;
    DOD3=DODdn2;
    ibatcAv1=IcAve;
    ibatdAv1=ibatdAv2;
end
